simulink model "usv_4dof_slidin"  (R2023b)
settings: Solver=VariableStepAuto  StartTime=0.0  StopTime=200  RelTol=1e-3
model workspace (MAT data in the model file):
  x0 = 0
settings Model: Creator=hw  LastModifiedBy=hw

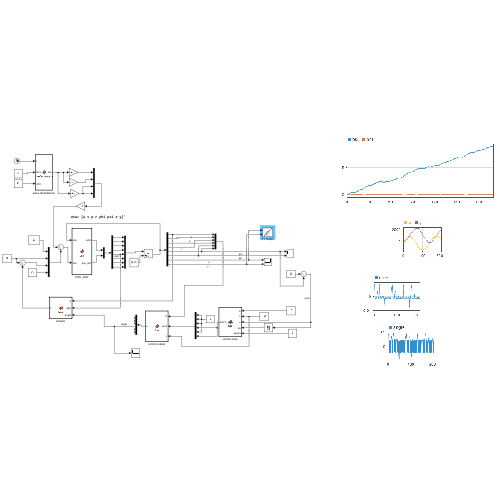
[thumbnail: Simulink's stored preview of the top-level diagram]
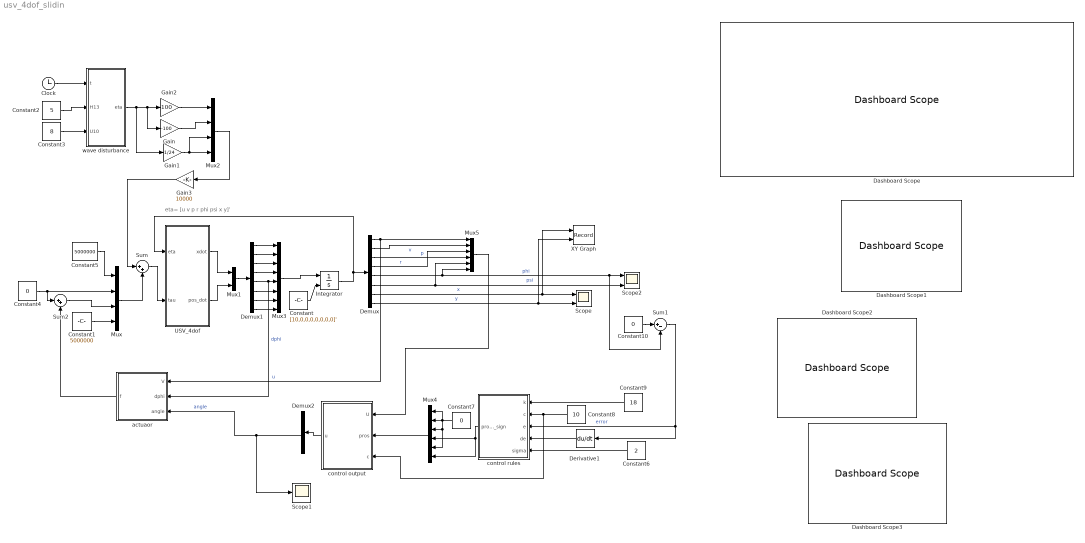
== system usv_4dof_slidin ==
  note: eta= [u v p r phi psi x y]'
  Clock : Clock
  Constant : Constant  Value=[10,0,0,0,0,0,0,0]'  VectorParams1D=off
  Constant1 : Constant  Value=5000000
  Constant10 : Constant  Value=0
  Constant2 : Constant  Value=5
  Constant3 : Constant  Value=8
  Constant4 : Constant  Value=0
  Constant5 : Constant  Value=5000000
  Constant6 : Constant  Value=2
  Constant7 : Constant  Value=0
  Constant8 : Constant  Value=10
  Constant9 : Constant  Value=18
  Dashboard Scope{,1..3} (4 alike) : DashboardScope
  Demux : Demux  Outputs=8
  Demux1 : Demux  Outputs=8
  Demux2 : Demux  Outputs=6
  Derivative1 : Derivative
  Gain : Gain  Gain=-100
  Gain1 : Gain  Gain=1/24
  Gain2 : Gain  Gain=100
  Gain3 : Gain  Gain=10000
  Integrator : Integrator  InitialConditionSource=external
  Mux : Mux
  Mux1 : Mux  Inputs=2
  Mux2 : Mux
  Mux3 : Mux  Inputs=8
  Mux4 : Mux  Inputs=6
  Mux5 : Mux  Inputs=6
  Scope : Scope  NumInputPorts=2
  Scope1 : Scope
  Scope2 : Scope  NumInputPorts=2
  Sum : Sum  Inputs=|++
  Sum1 : Sum  Inputs=|+-
  Sum2 : Sum  Inputs=|++
  USV_4dof : MATLAB Function  TreatAsAtomicUnit=on
  XY Graph : Record  FileSettingsInternal="{\"entries\":[{\"content\":{\"excelSettings\":{\"content\":{},\"type\":\"Streamout.ExcelSettings\"}},\"type\":\"Streamout.FileSettingStorage\",\"uuid\":\"\"}],\"packageUris\":[\"http:\\/\\/schema.mathworks.com\\/mf0\\/streamout_blocks\\/R2020a\"],\"version\":\"1.0\"}"  Layout=[1 1]  SignalsInternal="{\"entries\":[{\"content\":{\"signals\":[{\"content\":{\"blockPath\":[],\"dimensions\":[1,1],\"domain\":\"\",\"lineColor\":\"#a2142f\",\"plots\":[1],\"port\":1,\"sid\":[\"\"],\"signalID\":4332,\"signalName\":\"x\"},\"type\":\"RecordBlkView.Signal\",\"uuid\":\"\"},{\"content\":{\"blockPath\":[],\"dimensions\":[1,1],\"domain\":\"\",\"lineColor\":\"#139fff\",\"plots\":[1],\"port\":2,\"sid\":[\"\"],\"signalID\":4336,\"signalName\":\"y\"},\"type\":\"RecordBlkView.Signal\",\"uuid\":\"\"}]},\"type\":\"RecordBlkView.InputSignals\",\"uuid\":\"\"}],\"packageUris\":[\"http:\\/\\/schema.mathworks.com\\/mf0\\/streamout_blocks\\/R2020a\"],\"version\":\"1.0\"}"  VisualizationBindings="{\"xyplotplugin\":{\"info\":[{\"series\":[{\"bindingParametersList\":[{\"parameter\":\"X-Axis\",\"signalID\":4332,\"signalName\":\"x\"},{\"parameter\":\"Y-Axis\",\"signalID\":4336,\"signalName\":\"y\"}],\"seriesID\":54684}],\"subplotID\":1}]}}"  CompatibilityTag=XY
  actuaor : MATLAB Function  TreatAsAtomicUnit=on
  control output : MATLAB Function  TreatAsAtomicUnit=on
  control rules : MATLAB Function  TreatAsAtomicUnit=on
  wave disturbance : MATLAB Function  TreatAsAtomicUnit=on
  wires:
  USV_4dof/1(xdot) -> Mux1/1
  USV_4dof/2(pos_dot) -> Mux1/2
  Integrator/1 -> USV_4dof/1(eta), Demux/1
  Demux/7 -> Scope/1, XY Graph/1  "x"
  Demux/8 -> XY Graph/2, Scope/2  "y"
  Demux/5 -> Mux5/6, Sum1/2, Scope2/1  "phi"
  Demux/6 -> Mux5/5, Scope2/2  "psi"
  Demux/1 -> actuaor/1(V), Mux5/1  "u"
  Demux/2 -> Mux5/2  "v"
  Demux/3 -> Mux5/4  "p"
  Demux/4 -> Mux5/3  "r"
  Constant/1 -> Integrator/2
  Constant3/1 -> wave disturbance/3(U10)
  Clock/1 -> wave disturbance/1(t)
  wave disturbance/1(eta) -> Gain1/1, Gain/1, Gain2/1
  Constant2/1 -> wave disturbance/2(H13)
  Constant1/1 -> Mux/4
  Constant4/1 -> Sum2/1, Mux/2
  Constant5/1 -> Mux/1
  Gain/1 -> Mux2/2
  Gain2/1 -> Mux2/1
  Gain1/1 -> Mux2/3, Mux2/4
  Mux2/1 -> Gain3/1
  Demux1/1 -> Mux3/1
  Demux1/2 -> Mux3/2
  Demux1/3 -> Mux3/3
  Demux1/4 -> Mux3/4
  Demux1/5 -> actuaor/2(dphi), Mux3/5  "dphi"
  Demux1/6 -> Mux3/6
  Mux1/1 -> Demux1/1
  Mux3/1 -> Integrator/1
  Demux1/7 -> Mux3/7
  Demux1/8 -> Mux3/8
  Derivative1/1 -> control rules/4(de)
  Constant9/1 -> control rules/1(k)
  Mux4/1 -> control output/2(pros)
  Mux/1 -> Sum/2
  Sum/1 -> USV_4dof/2(tau)
  Mux5/1 -> control output/1(U)
  control output/1(u) -> Demux2/1
  Constant7/1 -> Mux4/1, Mux4/5, Mux4/3, Mux4/2
  control rules/1(prox1_sign) -> Mux4/6, Mux4/4
  Constant10/1 -> Sum1/1
  Sum1/1 -> Derivative1/1, control rules/3(e)  "error"
  Demux2/4 -> Scope1/1, actuaor/3(angle)  "angle"
  Sum2/1 -> Mux/3
  Constant8/1 -> control output/3(c), control rules/2(c)
  Constant6/1 -> control rules/5(sigma)
  actuaor/1(f) -> Sum2/2
  Gain3/1 -> Sum/1

== matlab function usv_4dof_slidin/USV_4dof ==
  data: eta input size=8*1; xdot output size=6*1; tau input; pos_dot output size=2*1
function [xdot,pos_dot] = usv(eta, tau)

% 线性化船舶模型
% Inputs:
% eta= [u v p r phi psi x y]'
% xdot= [du dv dp dr dphi dpsi]'
% pos_dot=[dx dy]'
% tau = [Xe Ye Ke Ne]' 
%

% where
% u     = surge velocity          (m/s)
% v     = sway velocity           (m/s)
% p     = roll velocity           (rad/s)
% r     = yaw velocity            (rad/s)
% phi   = roll angle              (rad)
% psi   = yaw angle               (rad)
%
% Xe is the surge external force (e.g. rudder and fin forces)
% Ye is the sway external force  
% Ke is the sway external force  
% Ne is the sway external force   

% Vessel Data
rho_water     =	1014.0;	        %	water density	[kg/m^3]	
rho_air		=	1.225	;	    %	air density		[kg/m^3]	
g				=	9.81;	        %	gravity constant	[m/s^2]	
deg2rad 		=	pi/180;	        %	degrees to radians	
rad2deg 		=	180/pi;	        %	rad to degrees		
ms2kt			=	3600/1852;	    % 	m/s to kt 			
kt2ms 		=	1852/3600;	    %	kt to m/s			
RPM2rads		=	2*pi/60;	    %	RPM to rad/s		
rads2RPM		=   60/(2*pi);	    %	rad/s to RPM		
HP2W			=	745.700;	    %	HP to Watt			


Lpp    =  51.5 ;                  % Length between perpendiculars垂直间长 [m]
B      =  8.6  ;                  % Beam over all 船宽 [m]
D	   =  2.3  ;                  % Draught吃水深度 [m]     

%Load condition (Modified by T.Perez)
disp   =  357.0;                   % Displacement 排水量 [m^3]
m      =  disp*rho_water;          % Mass [Kg]
Izz    =  47.934*10^6 ;            % Yaw Inertia偏航转动惯量
Ixx    =  2.3763*10^6 ;            % Roll Inertia横滚转动惯量
U_nom  =  8.0   ;	               % Speed nominal [m/sec]速度 (app 15kts) 
KM		=  4.47;	             %  [m] Transverse metacentre above keel 横倾复原力臂
KB		=  1.53;	             %  [m] Transverse centre of bouancy 浮心高度
gm 		=  1.1;	                 %  [m]	Transverse Metacenter 
bm 		=  KM - KB;
LCG       = 20.41 ;                % [m]	Longitudinal CG (from AP considered at the rudder stock)
VCG       = 3.36  ;                % [m]	Vertical  CG  above baseline
xG        = -3.38  ;               % coordinate of CG from the body fixed frame adopted for the PMM test  
zG  	    = -(VCG-D);          % coordinate of CG from the body fixed frame adopted for the PMM test  
m_xg	    = m * xG;
m_zg	    = m * zG;
Dp        = 1.6 ;                   % Propeller diameter [m]


% Data for surge equation 纵向（均为线性流体动力导数）
Xudot  	= -17400.0 ;  %-mx
Xuau     	= -1.96e+003 ;
Xvr    	=  0.33 * m ;
   
% Hydrodynamic coefficients in sway equation横向
Yvdot = -393000 ;  %-my
Ypdot = -296000 ; 
Yrdot = -1400000 ; %附加质量静距
Yauv  = -11800 ; 
Yur   =  131000 ; 
Yvav  = -3700 ; 
Yrar   =  0 ;
Yvar  = -794000 ; 
Yrav  = -182000 ; 
Ybauv =  10800 ; % Y_{\phi |v u|}
Ybaur =  251000 ; 
Ybuu  = -74 ; 


% Hydrodynamic coefficients in roll equation横摇水动力系数
Kvdot =  296000 ;
Kpdot = -774000 ;  %-Jxx
Krdot =  0 ;
Kauv  =  9260 ;
Kur   = -102000 ;
Kvav  =  29300 ;
Krar  =  0 ;
Kvar  =  621000 ;
Krav  =  142000 ;
Kbauv =  -8400 ;
Kbaur =  -196000 ;
Kbuu  =  -1180 ;
Kaup  =  -15500 ;
Kpap  =  -416000 ;
Kp    =  -500000 ;
Kb    =  0.776*m*g;
Kbbb  =  -0.325*m*g ;

% Hydrodynamic coefficients in yaw equation偏航水动力系数
Nvdot =  538000 ;   %-
Npdot =  0 ;
Nrdot = -38.7e6;    %jzz
Nauv  = -92000 ;
Naur  = -4710000 ;
Nvav  =  0 ;
Nrar  = -202000000 ;
Nvar  =  0 ;
Nrav  = -15600000 ;
Nbauv = -214000 ;
Nbuar = -4980000 ;
Nbuau = -8000 ;
%%%%%%%%%%%%%%%%%%%%%%%%%%%%%%%%%%%%%%%%%%%%%%%%%%%%%%%%%%%%%%%%%%%%%%%%%%%

% 定义输入
u   = eta(1);
v   = eta(2);
p  	= eta(3);   	
r  	= eta(4); 
b  	= eta(5); %phi roll 		
psi = eta(6);
x  	= eta(7);   	
y  	= eta(8); 
% 外部力与力矩
Xe  = tau(1);
Ye  = tau(2);
Ke  = tau(3);
Ne  = tau(4);

% Auxiliary variables辅助变量
au = abs(u);
av = abs(v); 
ar = abs(r); 
ap = abs(p); 
ab = abs(b);
L2 = Lpp^2; %参考面积？

% Total Mass Matrix 刚体质量矩阵
% x= [u v p r phi psi ]'
M =[ (m-Xudot)  0   0   0   0   0;
   0 (m-Yvdot) -(m*zG+Ypdot) (m*xG-Yrdot) 0 0;
   0 -(m*zG+Kvdot) (Ixx-Kpdot) -Krdot 0 0;
   0 (m*xG-Nvdot) -Npdot (Izz-Nrdot) 0 0;
   0 0 0 0 1 0; 
   0 0 0 0 0 1] ;
%转换矩阵
J=[cos(psi),-cos(b)*sin(psi);sin(psi),cos(b)*cos(psi)];
X=[u,v]';   
% Hydrodynamic forces without added mass terms(considered in the M matrix)
% 不考虑附加质量的水动力作用力 粘性流动动力（贵岛模型）
Xh  = Xuau*u*au+Xvr*v*r;

Yh = Yauv*au*v +  Yur*u*r + Yvav*v*av + Yvar*v*ar + Yrav*r*av + Ybauv*b*abs(u*v) + Ybaur*b*abs(u*r) + Ybuu*b*u^2;

Kh = Kauv*au*v +Kur*u*r + Kvav*v*av + Kvar*v*ar + Krav*r*av + Kbauv*b*abs(u*v) + Kbaur*b*abs(u*r) + Kbuu*b*u^2 +Kaup*au*p + Kpap*p*ap +Kp*p +Kbbb*b^3-(rho_water*g*gm*disp)*b;

Nh =Nauv*au*v + Naur*au*r +Nrar*r*ar + Nrav*r*av+Nbauv*b*abs(u*b) + Nbuar*b*u*ar + Nbuau*b*u*au;
 
% Rigid-body centripetal accelerations刚体运动产生的离心加速度影响
Xc =  m*(r*v+xG*r^2-zG*p*r);  
Yc = - m*u*r;
Kc =   m*zG*u*r;
Nc = - m*xG*u*r;

% Total forces
F1 = Xh+Xc+Xe;
F2 = Yh+Yc+Ye;
F4 = Kh+Kc+Ke;
F6 = Nh+Nc+Ne;

%运动学及动力学方程
pos_dot=J*X;
xdot = M\[F1; F2; F4; F6; p; r*cos(b)];

end

== matlab function usv_4dof_slidin/actuaor ==
  data: V input; dphi input; angle input size=1*1; f output size=1*1
function f  = top(V, dphi, angle)

d=2;
f=1/2*V^2*1025*10*0.87*(angle+dphi*d/V);
end

== matlab function usv_4dof_slidin/wave disturbance ==
  settings: updateMethod=DISCRETE
  data: t input; eta output; H13 input; U10 input
function eta = waveGeneration(t, H13, U10)
    % 此函数根据给定的有效波高和风速生成海浪信号
    % 常数定义
    g = 9.81; % 重力加速度, m/s^2
    alpha = 8.11e-3;
    beta = 3.11;
    
    % 风速对应的遭遇频率
    omega_e = 0.84 * (g / U10)^(1/3); % 峰值遭遇频率, rad/s

    % 频率范围和增量
    if H13 <= 2.5
        omegab=0.3;
        omegal =3.0;
        delta_omega = 0.1;
    elseif H13 <= 5.0
        omegab=0.25;
        omegal = 2.4;
        delta_omega = 0.08;
    else 
        omegab=0.1;
        omegal = 1.7;
        delta_omega = 0.06;
    end
    omega = omegab:delta_omega:omegal;

    % 能量密度谱 S(omega)
    S_omega = alpha * g^2 ./ omega.^5 .* exp(-beta ./ (H13^2 * omega.^4));
    % 振幅和相位
    a_omega = sqrt(2 * S_omega * delta_omega);
    phi = rand(1, length(omega)) * 2 * pi;
    % 海浪位移初始化
    eta = zeros(size(t));

    % 构建波形
    for i = 1:length(omega)
        eta = eta + a_omega(i) * cos(omega(i) * t + phi(i));
    end
end

== matlab function usv_4dof_slidin/control output ==
  data: U input; u output size=6*1; pros input; c input
function u= fcn(U,pros,c)
A = [-0.0115, 0.0692, -0.0054, 0,0,0 ;
     0, -0.0251, -3.4711, -0.1053, 0, -0.1931;
     0, -0.0011, -0.1080, 0.0114, 0, 0;
     0, 0.0023, -0.3293, -0.226, 0, -0.0741;
     0, 0, 1, 0, 0, 0 ;
     0, 0, 0, 1, 0, 0;]; %状态空间方程线性化A矩阵系数
E=diag([1,1,1,1,1,1]);
u=(-(A+E)*U-pros/c);

== matlab function usv_4dof_slidin/control rules ==
  data: k input; prox1_sign output; c input; e input; de input; sigma input
function prox1_sign= fcn(k, c,e,de,sigma)
s =c * e +de;
prox1_sign = (-1)* k * s - sigma * sign(s);
